simulink model "ex5_1"  (R2018b)
settings: Solver=VariableStepAuto  StartTime=0.0  StopTime=10  RelTol=1e-3
settings Model: Creator=HYJ  LastModifiedBy=HYJ

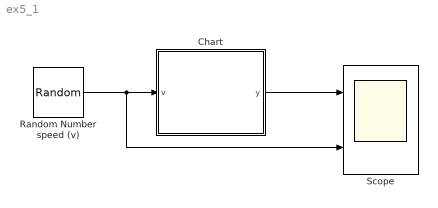
== system ex5_1 ==
  Chart : Stateflow chart  TreatAsAtomicUnit=on
  Random Number speed (v) : RandomNumber  Mean=85  Variance=20  SampleTime=0.1
  Scope : Scope  NumInputPorts=2
  wires:
  Chart/1(y) -> Scope/1
  Random Number speed (v)/1 -> Scope/2, Chart/1(v)

== stateflow chart ex5_1/Chart ==
  state LOW
    en: y=1;
  state MID
    en: y=2;
  state HIGH
    en: y=3;
  LOW -> HIGH [order 2] : [v>90]
  (default) -> LOW
  MID -> HIGH [order 1] : [v>90]
  LOW -> MID [order 1] : [v>80 && v<90]
  MID -> LOW [order 2] : [v<80]
  HIGH -> MID [order 1] : [v>80 && v<90]
  HIGH -> LOW [order 2] : [v<80]
  data: v input; y output
